simulink model "boucle_fermee_pi"  (R2014a)
settings: Solver=VariableStepAuto  StartTime=0.0  StopTime=1000  MaxStep=0.01  RelTol=1e-3
values from neighbouring files (symbols this model uses):
  k = 0.285    [parametres_tp2.m]
  Ti = 100    [parametres_tp2.m]
settings Model: Creator=12003927  LastModifiedBy=UTILISATEUR
settings DataIOCC: LimitDataPoints=off  SaveFormat=Dataset
settings OptimizationCC: LifeSpan=auto  SimCompilerOptimization=off
settings DebuggingCC: MergeDetectMultiDrivingBlocksExec=error  SolverPrmCheckMsg=none  FcnCallInpInsideContextMsg=error  FrameProcessingCompatibilityMsg=error  LibraryContextMissingDiagnostic=warning  SFUnexpectedBacktrackingDiag=error  SFNoUnconditionalDefaultTransitionDiag=error
settings HardwareCC: ProdBitPerPointer=64  ProdLargestAtomicFloat=Float  ProdIntDivRoundTo=Zero  ProdEndianess=LittleEndian  ProdWordSize=64  ProdHWDeviceType=Intel->x86-64 (Windows64)
settings ModelReferenceCC: PropagateSignalLabelsOutOfModel=on
settings SFSimCC: SimUseLocalCustomCode=on
settings RTWCC: RTWUseLocalCustomCode=on  RTWCompilerOptimization=off
settings GRTTargetCC: TargetLangStandard=C99 (ISO)  GeneratePreprocessorConditionals=Use local settings

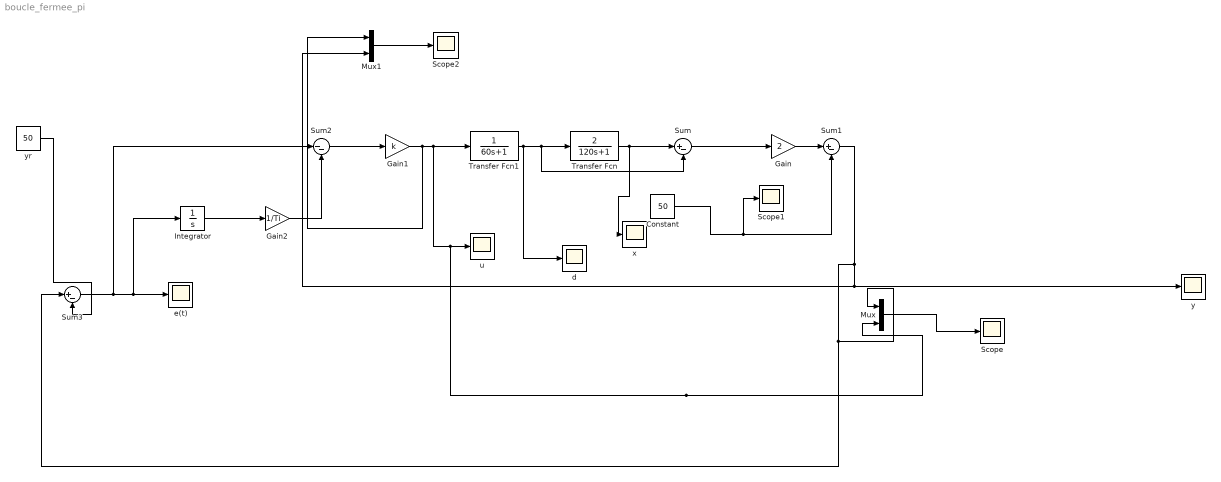
== system boucle_fermee_pi ==
  Constant : Constant  Value=50
  Gain : Gain  Gain=2
  Gain1 : Gain  Gain=k
  Gain2 : Gain  Gain=1/Ti
  Integrator : Integrator
  Mux : Mux  Inputs=2
  Mux1 : Mux  Inputs=2
  Scope : Scope
      settings: YMin=-500  YMax=500  SaveName=ScopeData2
  Scope1 : Scope
      settings: SaveName=ScopeData3
  Scope2 : Scope
      settings: SaveName=ScopeData4
  Sum : Sum  Inputs=|+-
  Sum1 : Sum  Inputs=|+-
  Sum2 : Sum  Inputs=|--
  Sum3 : Sum  Inputs=|+-
  Transfer Fcn : TransferFcn  Numerator=2  Denominator=[120 1]
  Transfer Fcn1 : TransferFcn  Denominator=[60 1]
  d : Scope
  e(t) : Scope
      settings: YMin=-120  YMax=120
  u : Scope
      settings: YMin=14.25  YMax=14.25
  x : Scope
  y : Scope
      settings: TimeRange=500  YMin=-100  YMax=200
  "yr " : Constant  Value=50
  wires:
  Transfer Fcn1/1 -> d/1, Sum/2, Transfer Fcn/1
  Sum/1 -> Gain/1
  Transfer Fcn/1 -> x/1, Sum/1
  Constant/1 -> Scope1/1, Sum1/2
  Gain/1 -> Sum1/1
  Sum2/1 -> Gain1/1
  Sum1/1 -> Mux/1, Sum3/1, y/1, Mux1/2
  Gain1/1 -> Mux1/1, Mux/2, u/1, Transfer Fcn1/1
  "yr "/1 -> Sum3/2
  Sum3/1 -> Sum2/1, Integrator/1, e(t)/1
  Mux/1 -> Scope/1
  Integrator/1 -> Gain2/1
  Gain2/1 -> Sum2/2
  Mux1/1 -> Scope2/1
